simulink model "DNN_x3D_M_2000iA900L_with_6_rev_21a"  (R2021a)
settings: Solver=VariableStepAuto  StartTime=0.0  StopTime=10.0  RelTol=1e-3
model workspace: external: MATLAB File /home/archistrax/Desktop/DNN/Simulink/Brazo robotico (2)/x3D_M_2000iA900L_OLGA_DataFile8.m (data not in the file)
values from neighbouring files (symbols this model uses):
  smiData = struct    [x3D_M_2000iA900L_OLGA_DataFile8.m]
undefined symbols (not defined in the file or in its folder): X, Y, Z
libraries: sm_lib x78, nesl_utility x31, pid_lib x15, dspmtrx3 x4
(part 1 of 4)
settings Model: Creator=olegfilatov  LastModifiedBy=archistrax
settings DataIOCC: InspectSignalLogs=on
settings HardwareCC: ProdBitPerLong=64  ProdHWDeviceType=Intel->x86-64 (Linux 64)

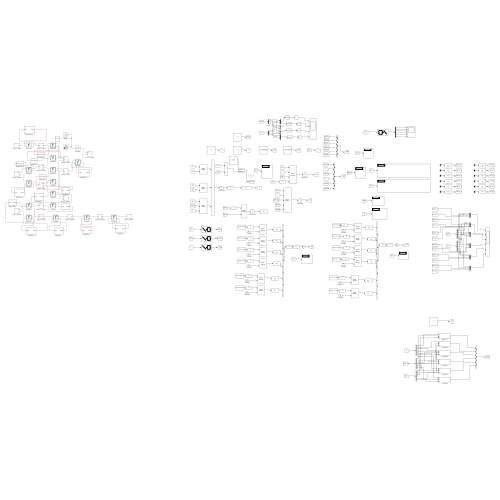
[thumbnail: Simulink's stored preview of the top-level diagram]
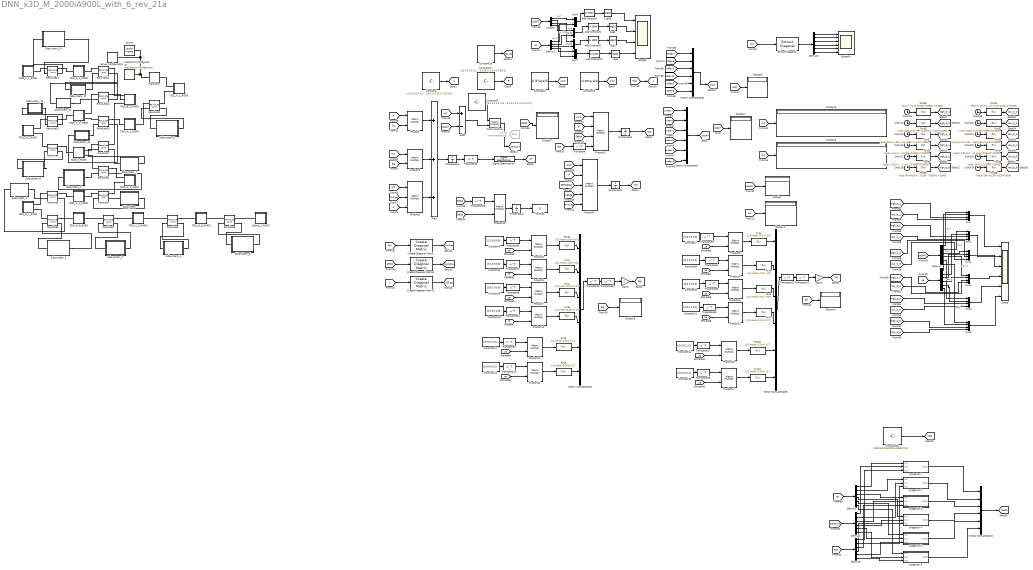
== system DNN_x3D_M_2000iA900L_with_6_rev_21a ==
  " " : Demux  Outputs=6
  Add : Sum  Inputs=+++
  Add Constant{,1..3} (4 alike) : Bias  Bias=1500
  Add1 : Sum  Inputs=+-
  Cabina_2_RIGID : Subsystem
  Clock{13..24} (12 alike) : Clock
  Constant : Constant  Value=[-25 0 0 0 0 0; 0 -35 0 0 0 0; 0 0 -15 0 0 0; 0 0 0 -19 0 0; 0 0 0 0 -20 0; 0 0 0 0 0 -20 ]*5.5  VectorParams1D=off
  Constant1 : Constant  Value=[5 0 0 0 0 0; 0 8 0 0 0 0; 0 0 10 0 0 0; 0 0 0 5 0 0; 0 0 0 0 5 0; 0 0 0 0 0 5 ]
  Constant10 : Constant  Value=[0 0 0 1 0 0]
  Constant11 : Constant  Value=[0 0 0 1 0 0]
  Constant12 : Constant  Value=[0 0 0 0 1 0]
  Constant13 : Constant  Value=[0 0 0 0 0 1]
  Constant14 : Constant  Value=[0 0 0 0 1 0]
  Constant15 : Constant  Value=[0 0 0 0 0 1]
  Constant16 : Constant  Value=[18 1 6 0.2; 1 25 5 0.4; 6 5 12 0.8; 0.2 0.4 0.8 22]*22  VectorParams1D=off
  Constant17 : Constant  Value=[25 0 0 0 0 0; 0 25 0 0 0 0; 0 0 10 0 0 0; 0 0 0 30 0 0; 0 0 0 0 25 0; 0 0 0 0 0 8]*15
  Constant18 : Constant  Value=[950;450;735;2200;40;650]*100
  Constant2 : Constant  Value=-0.8*eye(6)
  Constant3 : Constant  Value=-0.05*eye(6)
  Constant4 : Constant  Value=[1 0 0 0 0 0]
  Constant5 : Constant  Value=[0 1 0 0 0 0]
  Constant6 : Constant  Value=[0 0 1 0 0 0]
  Constant7 : Constant  Value=[1 0 0 0 0 0]
  Constant8 : Constant  Value=[0 1 0 0 0 0]
  Constant9 : Constant  Value=[0 0 1 0 0 0]
  Create Diagonal Matrix : dspmtrx3/Create Diagonal Matrix
      settings: SourceProductBaseCode=SL
  Create Diagonal Matrix1 : dspmtrx3/Create Diagonal Matrix
      settings: SourceProductBaseCode=SL
  Create Diagonal Matrix2 : dspmtrx3/Create Diagonal Matrix
      settings: SourceProductBaseCode=SL
  Demux{1,3..6} (5 alike) : Demux  Outputs=6
  Demux2 : Demux
  Display{,1..8} (9 alike) : Display
  Extract Diagonal : dspmtrx3/Extract Diagonal
      settings: SourceProductBaseCode=SL
  Fcn{1,3..5,11} (5 alike) : Fcn  Expr=2/(1+exp(-2*u))+0.5
  Fcn{2,6..10,12} (7 alike) : Fcn  Expr=1/(1+exp(-0.2*u))-0.7
  Fcn25 : Fcn  Expr=(exp(-u+0.1)+0.03+0.038*u)*10000
  Fcn26 : Fcn  Expr=(exp(-100*u+3)+0.31+0.0299*u-(0.007*u)^(0.5))*10000
  Fcn27 : Fcn  Expr=(exp(-0.2*u-1.05)*(sin(1.88*u)+2.5))*10000
  Fcn28 : Fcn  Expr=(exp(-u+0.1)+0.045+0.032*u)*10000
  Fcn29 : Fcn  Expr=(exp(-1.9*u+1.2)+0.2-0.008*u)*10000
  Fcn30 : Fcn  Expr=(exp(-8*u+6.5)+0.205 - 0.003*u)*10000
  Fcn31 : Fcn  Expr=(-exp(-2.2*u+1.2)-0.14+0.03*u)*10000
  Fcn32 : Fcn  Expr=(-exp(-100*u)-0.043+0.03*u)*10000
  Fcn33 : Fcn  Expr=-(exp(-0.2*u-0.5)*(1.8*cos(1.6*u)+2.8))*10000
  Fcn34 : Fcn  Expr=(-exp(-2.2*u+1.2)-0.14+0.03*u)*10000
  Fcn35 : Fcn  Expr=(-exp(-2*u+1.2)-0.42)*10000
  Fcn36 : Fcn  Expr=-(exp(-10*u+0.9)+0.53)*10000
  Gain3 : Gain
  Gain4 : Gain
  Goto31 : Goto  Commented=on  GotoTag=Delta  TagVisibility=global
  Log{1..3,10} (4 alike) : Math  Operator=log10  SaturateOnIntegerOverflow=on
  Matrix Multiply : Product  Multiplication=Matrix(*)
  MechanismConfiguration : sm_lib/Utilities/Mechanism Configuration  UniformGravity=Constant  GravityVector=[0 -9.80665 0]  GravityUnits=m/s^2  LinearizationDelta=0.001  JointModeTransitionNonlinearIterations=2
  Mux{,1..3,8..9} (6 alike) : Mux
  Mux{4..7} (4 alike) : Mux  Inputs=2
  Ozone-Gas1 : Integrator  InitialCondition=[0.2,0.1,0.01, 0.2,0.1,0.2;0.1,0.6,0.7,0.9,0.2,0.1;0.2,0.2,0.3,0.7,0.1,0.2; 0.2,0.9,0.7,0.5,0.2,0.1;0.1,0.2,0.3,0.4,0.2,0.2;0.4,0.3,0.2,0.1,0.1,0.2]
  Ozone-Gas2 : Integrator  InitialCondition=[0.2,0.1,0.01, 0.2,0.1,0.2;0.1,0.6,0.7,0.9,0.2,0.1;0.2,0.2,0.3,0.7,0.1,0.2; 0.2,0.9,0.7,0.5,0.2,0.1;0.1,0.2,0.3,0.4,0.2,0.2;0.4,0.3,0.2,0.1,0.1,0.2]
  Ozone-Gas3 : Integrator  InitialCondition=[0.2;0.3;0.1;0.3;0.2;0.2]*0.01
  Ozone-Gas4 : Integrator
  Product{,1,5..17} (15 alike) : Product  Multiplication=Matrix(*)
  Product2 : Product  Inputs=3  Multiplication=Matrix(*)
  Product3 : Product  Inputs=4  Multiplication=Matrix(*)
  Product4 : Product  Inputs=5  Multiplication=Matrix(*)
  Revolute : sm_lib/Joints/Revolute Joint  JointMode=Normal  SenseConstraintForce=off  SenseConstraintForceX=off  SenseConstraintForceY=off  SenseConstraintForceZ=off  SenseConstraintTorque=off  SenseConstraintTorqueX=off  SenseConstraintTorqueY=off  SenseConstraintTorqueZ=off  SenseTotalForce=off  SenseTotalForceX=off  SenseTotalForceY=off  SenseTotalForceZ=off  SenseTotalTorque=off  SenseTotalTorqueX=off  SenseTotalTorqueY=off  SenseTotalTorqueZ=off  CompositeWrenchDir=FollowerOnBase  CompositeWrenchFrame=BaseFrame  EquilibriumPosition=0  EquilibriumPositionUnits=deg  SpringStiffness=0  SpringStiffnessUnits=N*m/deg  DampingCoefficient=0  DampingCoefficientUnits=N*m/(deg/s)  TorqueActuationMode=InputTorque  MotionActuationMode=ComputedMotion  SensePosition=on  SenseVelocity=off  SenseAcceleration=off  SenseTorqueForce=off  SenseLowerLimitTorqueForce=off  SenseUpperLimitTorqueForce=off  LowerLimitSpecify=off  LowerLimitBound=-90  LowerLimitBoundUnits=deg  LowerLimitStiffness=1e4  LowerLimitStiffnessUnits=N*m/deg  LowerLimitDamping=10  LowerLimitDampingUnits=N*m/(deg/s)  LowerLimitTransitionRegionWidth=0.1  LowerLimitTransitionRegionWidthUnits=deg  UpperLimitSpecify=off  UpperLimitBound=90  UpperLimitBoundUnits=deg  UpperLimitStiffness=1e4  UpperLimitStiffnessUnits=N*m/deg  UpperLimitDamping=10  UpperLimitDampingUnits=N*m/(deg/s)  UpperLimitTransitionRegionWidth=0.1  UpperLimitTransitionRegionWidthUnits=deg  PositionTargetSpecify=on  PositionTargetPriority=Low  PositionTargetValue=smiData.RevoluteJoint(1).Rz.Pos  PositionTargetValueUnits=deg  VelocityTargetSpecify=off  VelocityTargetPriority=High  VelocityTargetValue=0  VelocityTargetValueUnits=deg/s
  Revolute1 : sm_lib/Joints/Revolute Joint  JointMode=Normal  SenseConstraintForce=off  SenseConstraintForceX=off  SenseConstraintForceY=off  SenseConstraintForceZ=off  SenseConstraintTorque=off  SenseConstraintTorqueX=off  SenseConstraintTorqueY=off  SenseConstraintTorqueZ=off  SenseTotalForce=off  SenseTotalForceX=off  SenseTotalForceY=off  SenseTotalForceZ=off  SenseTotalTorque=off  SenseTotalTorqueX=off  SenseTotalTorqueY=off  SenseTotalTorqueZ=off  CompositeWrenchDir=FollowerOnBase  CompositeWrenchFrame=BaseFrame  EquilibriumPosition=0  EquilibriumPositionUnits=deg  SpringStiffness=0  SpringStiffnessUnits=N*m/deg  DampingCoefficient=0  DampingCoefficientUnits=N*m/(deg/s)  TorqueActuationMode=InputTorque  MotionActuationMode=ComputedMotion  SensePosition=on  SenseVelocity=off  SenseAcceleration=off  SenseTorqueForce=off  SenseLowerLimitTorqueForce=off  SenseUpperLimitTorqueForce=off  LowerLimitSpecify=off  LowerLimitBound=-90  LowerLimitBoundUnits=deg  LowerLimitStiffness=1e4  LowerLimitStiffnessUnits=N*m/deg  LowerLimitDamping=10  LowerLimitDampingUnits=N*m/(deg/s)  LowerLimitTransitionRegionWidth=0.1  LowerLimitTransitionRegionWidthUnits=deg  UpperLimitSpecify=off  UpperLimitBound=90  UpperLimitBoundUnits=deg  UpperLimitStiffness=1e4  UpperLimitStiffnessUnits=N*m/deg  UpperLimitDamping=10  UpperLimitDampingUnits=N*m/(deg/s)  UpperLimitTransitionRegionWidth=0.1  UpperLimitTransitionRegionWidthUnits=deg  PositionTargetSpecify=on  PositionTargetPriority=Low  PositionTargetValue=smiData.RevoluteJoint(2).Rz.Pos  PositionTargetValueUnits=deg  VelocityTargetSpecify=off  VelocityTargetPriority=High  VelocityTargetValue=0  VelocityTargetValueUnits=deg/s
  Revolute10 : sm_lib/Joints/Revolute Joint  JointMode=Normal  SenseConstraintForce=off  SenseConstraintForceX=off  SenseConstraintForceY=off  SenseConstraintForceZ=off  SenseConstraintTorque=off  SenseConstraintTorqueX=off  SenseConstraintTorqueY=off  SenseConstraintTorqueZ=off  SenseTotalForce=off  SenseTotalForceX=off  SenseTotalForceY=off  SenseTotalForceZ=off  SenseTotalTorque=off  SenseTotalTorqueX=off  SenseTotalTorqueY=off  SenseTotalTorqueZ=off  CompositeWrenchDir=FollowerOnBase  CompositeWrenchFrame=BaseFrame  EquilibriumPosition=0  EquilibriumPositionUnits=deg  SpringStiffness=0  SpringStiffnessUnits=N*m/deg  DampingCoefficient=0  DampingCoefficientUnits=N*m/(deg/s)  TorqueActuationMode=InputTorque  MotionActuationMode=ComputedMotion  SensePosition=on  SenseVelocity=off  SenseAcceleration=off  SenseTorqueForce=off  SenseLowerLimitTorqueForce=off  SenseUpperLimitTorqueForce=off  LowerLimitSpecify=off  LowerLimitBound=-90  LowerLimitBoundUnits=deg  LowerLimitStiffness=1e4  LowerLimitStiffnessUnits=N*m/deg  LowerLimitDamping=10  LowerLimitDampingUnits=N*m/(deg/s)  LowerLimitTransitionRegionWidth=0.1  LowerLimitTransitionRegionWidthUnits=deg  UpperLimitSpecify=off  UpperLimitBound=90  UpperLimitBoundUnits=deg  UpperLimitStiffness=1e4  UpperLimitStiffnessUnits=N*m/deg  UpperLimitDamping=10  UpperLimitDampingUnits=N*m/(deg/s)  UpperLimitTransitionRegionWidth=0.1  UpperLimitTransitionRegionWidthUnits=deg  PositionTargetSpecify=on  PositionTargetPriority=Low  PositionTargetValue=smiData.RevoluteJoint(11).Rz.Pos  PositionTargetValueUnits=deg  VelocityTargetSpecify=off  VelocityTargetPriority=High  VelocityTargetValue=0  VelocityTargetValueUnits=deg/s
  Revolute11 : sm_lib/Joints/Revolute Joint  JointMode=Normal  SenseConstraintForce=off  SenseConstraintForceX=off  SenseConstraintForceY=off  SenseConstraintForceZ=off  SenseConstraintTorque=off  SenseConstraintTorqueX=off  SenseConstraintTorqueY=off  SenseConstraintTorqueZ=off  SenseTotalForce=off  SenseTotalForceX=off  SenseTotalForceY=off  SenseTotalForceZ=off  SenseTotalTorque=off  SenseTotalTorqueX=off  SenseTotalTorqueY=off  SenseTotalTorqueZ=off  CompositeWrenchDir=FollowerOnBase  CompositeWrenchFrame=BaseFrame  EquilibriumPosition=0  EquilibriumPositionUnits=deg  SpringStiffness=0  SpringStiffnessUnits=N*m/deg  DampingCoefficient=0  DampingCoefficientUnits=N*m/(deg/s)  TorqueActuationMode=InputTorque  MotionActuationMode=ComputedMotion  SensePosition=on  SenseVelocity=off  SenseAcceleration=off  SenseTorqueForce=off  SenseLowerLimitTorqueForce=off  SenseUpperLimitTorqueForce=off  LowerLimitSpecify=off  LowerLimitBound=-90  LowerLimitBoundUnits=deg  LowerLimitStiffness=1e4  LowerLimitStiffnessUnits=N*m/deg  LowerLimitDamping=10  LowerLimitDampingUnits=N*m/(deg/s)  LowerLimitTransitionRegionWidth=0.1  LowerLimitTransitionRegionWidthUnits=deg  UpperLimitSpecify=off  UpperLimitBound=90  UpperLimitBoundUnits=deg  UpperLimitStiffness=1e4  UpperLimitStiffnessUnits=N*m/deg  UpperLimitDamping=10  UpperLimitDampingUnits=N*m/(deg/s)  UpperLimitTransitionRegionWidth=0.1  UpperLimitTransitionRegionWidthUnits=deg  PositionTargetSpecify=on  PositionTargetPriority=Low  PositionTargetValue=smiData.RevoluteJoint(12).Rz.Pos  PositionTargetValueUnits=deg  VelocityTargetSpecify=off  VelocityTargetPriority=High  VelocityTargetValue=0  VelocityTargetValueUnits=deg/s
  Revolute12 : sm_lib/Joints/Revolute Joint  JointMode=Normal  SenseConstraintForce=off  SenseConstraintForceX=off  SenseConstraintForceY=off  SenseConstraintForceZ=off  SenseConstraintTorque=off  SenseConstraintTorqueX=off  SenseConstraintTorqueY=off  SenseConstraintTorqueZ=off  SenseTotalForce=off  SenseTotalForceX=off  SenseTotalForceY=off  SenseTotalForceZ=off  SenseTotalTorque=off  SenseTotalTorqueX=off  SenseTotalTorqueY=off  SenseTotalTorqueZ=off  CompositeWrenchDir=FollowerOnBase  CompositeWrenchFrame=BaseFrame  EquilibriumPosition=0  EquilibriumPositionUnits=deg  SpringStiffness=0  SpringStiffnessUnits=N*m/deg  DampingCoefficient=0  DampingCoefficientUnits=N*m/(deg/s)  TorqueActuationMode=InputTorque  MotionActuationMode=ComputedMotion  SensePosition=on  SenseVelocity=off  SenseAcceleration=off  SenseTorqueForce=off  SenseLowerLimitTorqueForce=off  SenseUpperLimitTorqueForce=off  LowerLimitSpecify=on  LowerLimitBound=-60  LowerLimitBoundUnits=deg  LowerLimitStiffness=1e4  LowerLimitStiffnessUnits=N*m/deg  LowerLimitDamping=10  LowerLimitDampingUnits=N*m/(deg/s)  LowerLimitTransitionRegionWidth=0.1  LowerLimitTransitionRegionWidthUnits=deg  UpperLimitSpecify=on  UpperLimitBound=100  UpperLimitBoundUnits=deg  UpperLimitStiffness=1e4  UpperLimitStiffnessUnits=N*m/deg  UpperLimitDamping=10  UpperLimitDampingUnits=N*m/(deg/s)  UpperLimitTransitionRegionWidth=0.1  UpperLimitTransitionRegionWidthUnits=deg  PositionTargetSpecify=on  PositionTargetPriority=Low  PositionTargetValue=smiData.RevoluteJoint(13).Rz.Pos  PositionTargetValueUnits=deg  VelocityTargetSpecify=off  VelocityTargetPriority=High  VelocityTargetValue=0  VelocityTargetValueUnits=deg/s
  Revolute13 : sm_lib/Joints/Revolute Joint  JointMode=Normal  SenseConstraintForce=off  SenseConstraintForceX=off  SenseConstraintForceY=off  SenseConstraintForceZ=off  SenseConstraintTorque=off  SenseConstraintTorqueX=off  SenseConstraintTorqueY=off  SenseConstraintTorqueZ=off  SenseTotalForce=off  SenseTotalForceX=off  SenseTotalForceY=off  SenseTotalForceZ=off  SenseTotalTorque=off  SenseTotalTorqueX=off  SenseTotalTorqueY=off  SenseTotalTorqueZ=off  CompositeWrenchDir=FollowerOnBase  CompositeWrenchFrame=BaseFrame  EquilibriumPosition=0  EquilibriumPositionUnits=deg  SpringStiffness=0  SpringStiffnessUnits=N*m/deg  DampingCoefficient=0  DampingCoefficientUnits=N*m/(deg/s)  TorqueActuationMode=InputTorque  MotionActuationMode=ComputedMotion  SensePosition=on  SenseVelocity=off  SenseAcceleration=off  SenseTorqueForce=off  SenseLowerLimitTorqueForce=off  SenseUpperLimitTorqueForce=off  LowerLimitSpecify=off  LowerLimitBound=-90  LowerLimitBoundUnits=deg  LowerLimitStiffness=1e4  LowerLimitStiffnessUnits=N*m/deg  LowerLimitDamping=10  LowerLimitDampingUnits=N*m/(deg/s)  LowerLimitTransitionRegionWidth=0.1  LowerLimitTransitionRegionWidthUnits=deg  UpperLimitSpecify=off  UpperLimitBound=90  UpperLimitBoundUnits=deg  UpperLimitStiffness=1e4  UpperLimitStiffnessUnits=N*m/deg  UpperLimitDamping=10  UpperLimitDampingUnits=N*m/(deg/s)  UpperLimitTransitionRegionWidth=0.1  UpperLimitTransitionRegionWidthUnits=deg  PositionTargetSpecify=on  PositionTargetPriority=Low  PositionTargetValue=smiData.RevoluteJoint(14).Rz.Pos  PositionTargetValueUnits=deg  VelocityTargetSpecify=off  VelocityTargetPriority=High  VelocityTargetValue=0  VelocityTargetValueUnits=deg/s
  Revolute14 : sm_lib/Joints/Revolute Joint  JointMode=Normal  SenseConstraintForce=off  SenseConstraintForceX=off  SenseConstraintForceY=off  SenseConstraintForceZ=off  SenseConstraintTorque=off  SenseConstraintTorqueX=off  SenseConstraintTorqueY=off  SenseConstraintTorqueZ=off  SenseTotalForce=off  SenseTotalForceX=off  SenseTotalForceY=off  SenseTotalForceZ=off  SenseTotalTorque=off  SenseTotalTorqueX=off  SenseTotalTorqueY=off  SenseTotalTorqueZ=off  CompositeWrenchDir=FollowerOnBase  CompositeWrenchFrame=BaseFrame  EquilibriumPosition=0  EquilibriumPositionUnits=deg  SpringStiffness=0  SpringStiffnessUnits=N*m/deg  DampingCoefficient=0  DampingCoefficientUnits=N*m/(deg/s)  TorqueActuationMode=InputTorque  MotionActuationMode=ComputedMotion  SensePosition=on  SenseVelocity=off  SenseAcceleration=off  SenseTorqueForce=off  SenseLowerLimitTorqueForce=off  SenseUpperLimitTorqueForce=off  LowerLimitSpecify=off  LowerLimitBound=-90  LowerLimitBoundUnits=deg  LowerLimitStiffness=1e4  LowerLimitStiffnessUnits=N*m/deg  LowerLimitDamping=10  LowerLimitDampingUnits=N*m/(deg/s)  LowerLimitTransitionRegionWidth=0.1  LowerLimitTransitionRegionWidthUnits=deg  UpperLimitSpecify=off  UpperLimitBound=90  UpperLimitBoundUnits=deg  UpperLimitStiffness=1e4  UpperLimitStiffnessUnits=N*m/deg  UpperLimitDamping=10  UpperLimitDampingUnits=N*m/(deg/s)  UpperLimitTransitionRegionWidth=0.1  UpperLimitTransitionRegionWidthUnits=deg  PositionTargetSpecify=on  PositionTargetPriority=Low  PositionTargetValue=smiData.RevoluteJoint(15).Rz.Pos  PositionTargetValueUnits=deg  VelocityTargetSpecify=off  VelocityTargetPriority=High  VelocityTargetValue=0  VelocityTargetValueUnits=deg/s
  Revolute2 : sm_lib/Joints/Revolute Joint  JointMode=Normal  SenseConstraintForce=off  SenseConstraintForceX=off  SenseConstraintForceY=off  SenseConstraintForceZ=off  SenseConstraintTorque=off  SenseConstraintTorqueX=off  SenseConstraintTorqueY=off  SenseConstraintTorqueZ=off  SenseTotalForce=off  SenseTotalForceX=off  SenseTotalForceY=off  SenseTotalForceZ=off  SenseTotalTorque=off  SenseTotalTorqueX=off  SenseTotalTorqueY=off  SenseTotalTorqueZ=off  CompositeWrenchDir=FollowerOnBase  CompositeWrenchFrame=BaseFrame  EquilibriumPosition=0  EquilibriumPositionUnits=deg  SpringStiffness=0  SpringStiffnessUnits=N*m/deg  DampingCoefficient=0  DampingCoefficientUnits=N*m/(deg/s)  TorqueActuationMode=InputTorque  MotionActuationMode=ComputedMotion  SensePosition=on  SenseVelocity=off  SenseAcceleration=off  SenseTorqueForce=off  SenseLowerLimitTorqueForce=off  SenseUpperLimitTorqueForce=off  LowerLimitSpecify=on  LowerLimitBound=-120  LowerLimitBoundUnits=deg  LowerLimitStiffness=1e4  LowerLimitStiffnessUnits=N*m/deg  LowerLimitDamping=10  LowerLimitDampingUnits=N*m/(deg/s)  LowerLimitTransitionRegionWidth=0.1  LowerLimitTransitionRegionWidthUnits=deg  UpperLimitSpecify=on  UpperLimitBound=120  UpperLimitBoundUnits=deg  UpperLimitStiffness=1e4  UpperLimitStiffnessUnits=N*m/deg  UpperLimitDamping=10  UpperLimitDampingUnits=N*m/(deg/s)  UpperLimitTransitionRegionWidth=0.1  UpperLimitTransitionRegionWidthUnits=deg  PositionTargetSpecify=on  PositionTargetPriority=Low  PositionTargetValue=smiData.RevoluteJoint(3).Rz.Pos  PositionTargetValueUnits=deg  VelocityTargetSpecify=off  VelocityTargetPriority=High  VelocityTargetValue=0  VelocityTargetValueUnits=deg/s
  Revolute3 : sm_lib/Joints/Revolute Joint  JointMode=Normal  SenseConstraintForce=off  SenseConstraintForceX=off  SenseConstraintForceY=off  SenseConstraintForceZ=off  SenseConstraintTorque=off  SenseConstraintTorqueX=off  SenseConstraintTorqueY=off  SenseConstraintTorqueZ=off  SenseTotalForce=off  SenseTotalForceX=off  SenseTotalForceY=off  SenseTotalForceZ=off  SenseTotalTorque=off  SenseTotalTorqueX=off  SenseTotalTorqueY=off  SenseTotalTorqueZ=off  CompositeWrenchDir=FollowerOnBase  CompositeWrenchFrame=BaseFrame  EquilibriumPosition=0  EquilibriumPositionUnits=deg  SpringStiffness=0  SpringStiffnessUnits=N*m/deg  DampingCoefficient=0  DampingCoefficientUnits=N*m/(deg/s)  TorqueActuationMode=InputTorque  MotionActuationMode=ComputedMotion  SensePosition=on  SenseVelocity=off  SenseAcceleration=off  SenseTorqueForce=off  SenseLowerLimitTorqueForce=off  SenseUpperLimitTorqueForce=off  LowerLimitSpecify=on  LowerLimitBound=-360  LowerLimitBoundUnits=deg  LowerLimitStiffness=1e4  LowerLimitStiffnessUnits=N*m/deg  LowerLimitDamping=10  LowerLimitDampingUnits=N*m/(deg/s)  LowerLimitTransitionRegionWidth=0.1  LowerLimitTransitionRegionWidthUnits=deg  UpperLimitSpecify=on  UpperLimitBound=360  UpperLimitBoundUnits=deg  UpperLimitStiffness=1e4  UpperLimitStiffnessUnits=N*m/deg  UpperLimitDamping=10  UpperLimitDampingUnits=N*m/(deg/s)  UpperLimitTransitionRegionWidth=0.1  UpperLimitTransitionRegionWidthUnits=deg  PositionTargetSpecify=on  PositionTargetPriority=Low  PositionTargetValue=smiData.RevoluteJoint(4).Rz.Pos  PositionTargetValueUnits=deg  VelocityTargetSpecify=off  VelocityTargetPriority=High  VelocityTargetValue=0  VelocityTargetValueUnits=deg/s
  Revolute4 : sm_lib/Joints/Revolute Joint  JointMode=Normal  SenseConstraintForce=off  SenseConstraintForceX=off  SenseConstraintForceY=off  SenseConstraintForceZ=off  SenseConstraintTorque=off  SenseConstraintTorqueX=off  SenseConstraintTorqueY=off  SenseConstraintTorqueZ=off  SenseTotalForce=off  SenseTotalForceX=off  SenseTotalForceY=off  SenseTotalForceZ=off  SenseTotalTorque=off  SenseTotalTorqueX=off  SenseTotalTorqueY=off  SenseTotalTorqueZ=off  CompositeWrenchDir=FollowerOnBase  CompositeWrenchFrame=BaseFrame  EquilibriumPosition=0  EquilibriumPositionUnits=deg  SpringStiffness=0  SpringStiffnessUnits=N*m/deg  DampingCoefficient=0  DampingCoefficientUnits=N*m/(deg/s)  TorqueActuationMode=InputTorque  MotionActuationMode=ComputedMotion  SensePosition=on  SenseVelocity=off  SenseAcceleration=off  SenseTorqueForce=off  SenseLowerLimitTorqueForce=off  SenseUpperLimitTorqueForce=off  LowerLimitSpecify=off  LowerLimitBound=-90  LowerLimitBoundUnits=deg  LowerLimitStiffness=1e4  LowerLimitStiffnessUnits=N*m/deg  LowerLimitDamping=10  LowerLimitDampingUnits=N*m/(deg/s)  LowerLimitTransitionRegionWidth=0.1  LowerLimitTransitionRegionWidthUnits=deg  UpperLimitSpecify=off  UpperLimitBound=90  UpperLimitBoundUnits=deg  UpperLimitStiffness=1e4  UpperLimitStiffnessUnits=N*m/deg  UpperLimitDamping=10  UpperLimitDampingUnits=N*m/(deg/s)  UpperLimitTransitionRegionWidth=0.1  UpperLimitTransitionRegionWidthUnits=deg  PositionTargetSpecify=on  PositionTargetPriority=Low  PositionTargetValue=smiData.RevoluteJoint(5).Rz.Pos  PositionTargetValueUnits=deg  VelocityTargetSpecify=off  VelocityTargetPriority=High  VelocityTargetValue=0  VelocityTargetValueUnits=deg/s
  Revolute5 : sm_lib/Joints/Revolute Joint  JointMode=Normal  SenseConstraintForce=off  SenseConstraintForceX=off  SenseConstraintForceY=off  SenseConstraintForceZ=off  SenseConstraintTorque=off  SenseConstraintTorqueX=off  SenseConstraintTorqueY=off  SenseConstraintTorqueZ=off  SenseTotalForce=off  SenseTotalForceX=off  SenseTotalForceY=off  SenseTotalForceZ=off  SenseTotalTorque=off  SenseTotalTorqueX=off  SenseTotalTorqueY=off  SenseTotalTorqueZ=off  CompositeWrenchDir=FollowerOnBase  CompositeWrenchFrame=BaseFrame  EquilibriumPosition=0  EquilibriumPositionUnits=deg  SpringStiffness=0  SpringStiffnessUnits=N*m/deg  DampingCoefficient=0  DampingCoefficientUnits=N*m/(deg/s)  TorqueActuationMode=InputTorque  MotionActuationMode=ComputedMotion  SensePosition=on  SenseVelocity=off  SenseAcceleration=off  SenseTorqueForce=off  SenseLowerLimitTorqueForce=off  SenseUpperLimitTorqueForce=off  LowerLimitSpecify=off  LowerLimitBound=-90  LowerLimitBoundUnits=deg  LowerLimitStiffness=1e4  LowerLimitStiffnessUnits=N*m/deg  LowerLimitDamping=10  LowerLimitDampingUnits=N*m/(deg/s)  LowerLimitTransitionRegionWidth=0.1  LowerLimitTransitionRegionWidthUnits=deg  UpperLimitSpecify=off  UpperLimitBound=90  UpperLimitBoundUnits=deg  UpperLimitStiffness=1e4  UpperLimitStiffnessUnits=N*m/deg  UpperLimitDamping=10  UpperLimitDampingUnits=N*m/(deg/s)  UpperLimitTransitionRegionWidth=0.1  UpperLimitTransitionRegionWidthUnits=deg  PositionTargetSpecify=on  PositionTargetPriority=Low  PositionTargetValue=smiData.RevoluteJoint(6).Rz.Pos  PositionTargetValueUnits=deg  VelocityTargetSpecify=off  VelocityTargetPriority=High  VelocityTargetValue=0  VelocityTargetValueUnits=deg/s
  Revolute6 : sm_lib/Joints/Revolute Joint  JointMode=Normal  SenseConstraintForce=off  SenseConstraintForceX=off  SenseConstraintForceY=off  SenseConstraintForceZ=off  SenseConstraintTorque=off  SenseConstraintTorqueX=off  SenseConstraintTorqueY=off  SenseConstraintTorqueZ=off  SenseTotalForce=off  SenseTotalForceX=off  SenseTotalForceY=off  SenseTotalForceZ=off  SenseTotalTorque=off  SenseTotalTorqueX=off  SenseTotalTorqueY=off  SenseTotalTorqueZ=off  CompositeWrenchDir=FollowerOnBase  CompositeWrenchFrame=BaseFrame  EquilibriumPosition=0  EquilibriumPositionUnits=deg  SpringStiffness=0  SpringStiffnessUnits=N*m/deg  DampingCoefficient=0  DampingCoefficientUnits=N*m/(deg/s)  TorqueActuationMode=InputTorque  MotionActuationMode=ComputedMotion  SensePosition=on  SenseVelocity=off  SenseAcceleration=off  SenseTorqueForce=off  SenseLowerLimitTorqueForce=off  SenseUpperLimitTorqueForce=off  LowerLimitSpecify=on  LowerLimitBound=-360  LowerLimitBoundUnits=deg  LowerLimitStiffness=1e4  LowerLimitStiffnessUnits=N*m/deg  LowerLimitDamping=10  LowerLimitDampingUnits=N*m/(deg/s)  LowerLimitTransitionRegionWidth=0.1  LowerLimitTransitionRegionWidthUnits=deg  UpperLimitSpecify=on  UpperLimitBound=360  UpperLimitBoundUnits=deg  UpperLimitStiffness=1e4  UpperLimitStiffnessUnits=N*m/deg  UpperLimitDamping=10  UpperLimitDampingUnits=N*m/(deg/s)  UpperLimitTransitionRegionWidth=0.1  UpperLimitTransitionRegionWidthUnits=deg  PositionTargetSpecify=on  PositionTargetPriority=Low  PositionTargetValue=smiData.RevoluteJoint(7).Rz.Pos  PositionTargetValueUnits=deg  VelocityTargetSpecify=off  VelocityTargetPriority=High  VelocityTargetValue=0  VelocityTargetValueUnits=deg/s
  Revolute7 : sm_lib/Joints/Revolute Joint  JointMode=Normal  SenseConstraintForce=off  SenseConstraintForceX=off  SenseConstraintForceY=off  SenseConstraintForceZ=off  SenseConstraintTorque=off  SenseConstraintTorqueX=off  SenseConstraintTorqueY=off  SenseConstraintTorqueZ=off  SenseTotalForce=off  SenseTotalForceX=off  SenseTotalForceY=off  SenseTotalForceZ=off  SenseTotalTorque=off  SenseTotalTorqueX=off  SenseTotalTorqueY=off  SenseTotalTorqueZ=off  CompositeWrenchDir=FollowerOnBase  CompositeWrenchFrame=BaseFrame  EquilibriumPosition=0  EquilibriumPositionUnits=deg  SpringStiffness=0  SpringStiffnessUnits=N*m/deg  DampingCoefficient=0  DampingCoefficientUnits=N*m/(deg/s)  TorqueActuationMode=InputTorque  MotionActuationMode=ComputedMotion  SensePosition=on  SenseVelocity=off  SenseAcceleration=off  SenseTorqueForce=off  SenseLowerLimitTorqueForce=off  SenseUpperLimitTorqueForce=off  LowerLimitSpecify=on  LowerLimitBound=-130  LowerLimitBoundUnits=deg  LowerLimitStiffness=1e4  LowerLimitStiffnessUnits=N*m/deg  LowerLimitDamping=10  LowerLimitDampingUnits=N*m/(deg/s)  LowerLimitTransitionRegionWidth=0.1  LowerLimitTransitionRegionWidthUnits=deg  UpperLimitSpecify=on  UpperLimitBound=35  UpperLimitBoundUnits=deg  UpperLimitStiffness=1e4  UpperLimitStiffnessUnits=N*m/deg  UpperLimitDamping=10  UpperLimitDampingUnits=N*m/(deg/s)  UpperLimitTransitionRegionWidth=0.1  UpperLimitTransitionRegionWidthUnits=deg  PositionTargetSpecify=on  PositionTargetPriority=Low  PositionTargetValue=smiData.RevoluteJoint(8).Rz.Pos  PositionTargetValueUnits=deg  VelocityTargetSpecify=off  VelocityTargetPriority=High  VelocityTargetValue=0  VelocityTargetValueUnits=deg/s
  Revolute8 : sm_lib/Joints/Revolute Joint  JointMode=Normal  SenseConstraintForce=off  SenseConstraintForceX=off  SenseConstraintForceY=off  SenseConstraintForceZ=off  SenseConstraintTorque=off  SenseConstraintTorqueX=off  SenseConstraintTorqueY=off  SenseConstraintTorqueZ=off  SenseTotalForce=off  SenseTotalForceX=off  SenseTotalForceY=off  SenseTotalForceZ=off  SenseTotalTorque=off  SenseTotalTorqueX=off  SenseTotalTorqueY=off  SenseTotalTorqueZ=off  CompositeWrenchDir=FollowerOnBase  CompositeWrenchFrame=BaseFrame  EquilibriumPosition=0  EquilibriumPositionUnits=deg  SpringStiffness=0  SpringStiffnessUnits=N*m/deg  DampingCoefficient=0  DampingCoefficientUnits=N*m/(deg/s)  TorqueActuationMode=InputTorque  MotionActuationMode=ComputedMotion  SensePosition=on  SenseVelocity=off  SenseAcceleration=off  SenseTorqueForce=off  SenseLowerLimitTorqueForce=off  SenseUpperLimitTorqueForce=off  LowerLimitSpecify=off  LowerLimitBound=-90  LowerLimitBoundUnits=deg  LowerLimitStiffness=1e4  LowerLimitStiffnessUnits=N*m/deg  LowerLimitDamping=10  LowerLimitDampingUnits=N*m/(deg/s)  LowerLimitTransitionRegionWidth=0.1  LowerLimitTransitionRegionWidthUnits=deg  UpperLimitSpecify=off  UpperLimitBound=90  UpperLimitBoundUnits=deg  UpperLimitStiffness=1e4  UpperLimitStiffnessUnits=N*m/deg  UpperLimitDamping=10  UpperLimitDampingUnits=N*m/(deg/s)  UpperLimitTransitionRegionWidth=0.1  UpperLimitTransitionRegionWidthUnits=deg  PositionTargetSpecify=off  PositionTargetPriority=High  PositionTargetValue=0  PositionTargetValueUnits=deg  VelocityTargetSpecify=off  VelocityTargetPriority=High  VelocityTargetValue=0  VelocityTargetValueUnits=deg/s
  Revolute9 : sm_lib/Joints/Revolute Joint  JointMode=Normal  SenseConstraintForce=off  SenseConstraintForceX=off  SenseConstraintForceY=off  SenseConstraintForceZ=off  SenseConstraintTorque=off  SenseConstraintTorqueX=off  SenseConstraintTorqueY=off  SenseConstraintTorqueZ=off  SenseTotalForce=off  SenseTotalForceX=off  SenseTotalForceY=off  SenseTotalForceZ=off  SenseTotalTorque=off  SenseTotalTorqueX=off  SenseTotalTorqueY=off  SenseTotalTorqueZ=off  CompositeWrenchDir=FollowerOnBase  CompositeWrenchFrame=BaseFrame  EquilibriumPosition=0  EquilibriumPositionUnits=deg  SpringStiffness=0  SpringStiffnessUnits=N*m/deg  DampingCoefficient=0  DampingCoefficientUnits=N*m/(deg/s)  TorqueActuationMode=InputTorque  MotionActuationMode=ComputedMotion  SensePosition=on  SenseVelocity=off  SenseAcceleration=off  SenseTorqueForce=off  SenseLowerLimitTorqueForce=off  SenseUpperLimitTorqueForce=off  LowerLimitSpecify=on  LowerLimitBound=-165  LowerLimitBoundUnits=deg  LowerLimitStiffness=1e4  LowerLimitStiffnessUnits=N*m/deg  LowerLimitDamping=10  LowerLimitDampingUnits=N*m/(deg/s)  LowerLimitTransitionRegionWidth=0.1  LowerLimitTransitionRegionWidthUnits=deg  UpperLimitSpecify=on  UpperLimitBound=165  UpperLimitBoundUnits=deg  UpperLimitStiffness=1e4  UpperLimitStiffnessUnits=N*m/deg  UpperLimitDamping=10  UpperLimitDampingUnits=N*m/(deg/s)  UpperLimitTransitionRegionWidth=0.1  UpperLimitTransitionRegionWidthUnits=deg  PositionTargetSpecify=on  PositionTargetPriority=Low  PositionTargetValue=smiData.RevoluteJoint(10).Rz.Pos  PositionTargetValueUnits=deg  VelocityTargetSpecify=off  VelocityTargetPriority=High  VelocityTargetValue=0  VelocityTargetValueUnits=deg/s
  Scope : Scope  NumInputPorts=6
  Scope1 : Scope  NumInputPorts=4
  Scope14 : Scope  NumInputPorts=6
  Signal Specification : SignalSpecification  Dimensions=6
  Solver Configuration : nesl_utility/Solver Configuration  PhysicalDomain=network_engine_domain  SubClassName=solver  LeftPortType=input  RightPortType=generic  Tones=[]  Harmonics=[]  SimulateNoise=off  Profile=off  UseLocalSampling=off  EnableSwitchedLinearOptims=on  FrequencyDomain=off  UseCCode=off  RelTol=0.001  AbsTol=1e-06  MinStep=1e-09  ToWorkspace=off  RevertToSquareIcSolve=off  NumHomotopyIterations=100  PhasorMode=off  PhasorModeNumHarmonics=1  IndexReductionMethod=DerivativeReplacement  DoDC=off  ResidualTolerance=1e-09  UseLocalSolver=off  LocalSolverChoice=NE_BACKWARD_EULER_ADVANCER  LocalSolverSampleTime=0.001  DoFixedCost=off  MaxNonlinIter=3  MaxModeIter=2  ComputeImpulses=off  ImpulseIterations=2  LinearAlgebra=auto  LinearAlgebraNumThread=0  EquationFormulation=NE_TIME_EF  DelaysMemoryBudget=1024  AutomaticFiltering=on  FilteringTimeConstant=0.001  PartitionStorageMethod=AS_NEEDED  PartitionMemoryBudget=1024  PartitionMethod=ROBUST
      settings: SourceProductBaseCode=SS,PW,VE
  Subsystem : Subsystem
  Subsystem_1 : Subsystem
  Subsystem_10 : Subsystem
  Subsystem_11 : Subsystem
  Subsystem_12 : Subsystem
  Subsystem_13 : Subsystem
  Subsystem_14 : Subsystem
  Subsystem_2 : Subsystem
  Subsystem_3 : Subsystem
  Subsystem_4 : Subsystem
  Subsystem_5 : Subsystem
  Subsystem_6 : Subsystem
  Subsystem_7 : Subsystem
  Subsystem_8 : Subsystem
  Subsystem_9 : Subsystem
  T201_A_1_RIGID : Subsystem
  T301_A_1_RIGID : Subsystem
  T301_B_1_RIGID : Subsystem
  T301_D_1_RIGID : Subsystem
  T301_E_1_RIGID : Subsystem
  T301_F_1_RIGID : Subsystem
  T303_C_1_RIGID : Subsystem
  T403_1_RIGID : Subsystem
  T501_A_1_RIGID : Subsystem
  T501_A_6_RIGID : Subsystem
  T501_C_1_RIGID : Subsystem
  T501_C_6_RIGID : Subsystem
  T501_D_1_RIGID : Subsystem
  T501_D_6_RIGID : Subsystem
  To File4 : ToFile  Filename=Q  MatrixName=Q  SaveFormat=Timeseries
  Transform : sm_lib/Frames and Transforms/Rigid Transform  TranslationMethod=Cartesian  TranslationStandardOffset=0  TranslationLengthUnit=mm  TranslationStandardAxis=+Z  TranslationCartesianOffset=smiData.RigidTransform(31).translation  TranslationROffset=0  TranslationROffsetUnits=m  TranslationZOffset=0  TranslationZOffsetUnits=m  TranslationThetaOffset=0  TranslationThetaOffsetUnits=deg  RotationMethod=ArbitraryAxis  RotationAngleUnits=rad  RotationStandardAxis=+Z  RotationAngle=smiData.RigidTransform(31).angle  RotationArbitraryAxis=smiData.RigidTransform(31).axis  FollAlignAxisA=+X  BaseAlignAxisA=+Y  FollAlignAxisB=+Y  BaseAlignAxisB=+Z  RotationSequenceAxes=FollowerAxes  RotationSequence=XYX  RotationSequenceAngles=[0 0 0]  RotationSequenceAnglesUnits=deg  RotationMatrix=[1 0 0; 0 1 0; 0 0 1]
  Transpose{,1..18} (19 alike) : Math  Operator=transpose  SignedPower=on  SaturateOnIntegerOverflow=on
  Vector Concatenate{,1..4} (5 alike) : Concatenate  NumInputs=6
  World : sm_lib/Frames and Transforms/World Frame
  outAll1 : Demux
  progector 2 : Subsystem
  progector 3 : Subsystem
  progector 4 : Subsystem
  progector 5 : Subsystem
  progector 6 : Subsystem
  projector 1 : Subsystem
  tag scope: A=global, Delta=global, DeltaDiag=global, Delta_old=global, P=global, Phi=global, PhiDiag=global, Sig=global, UDiag=global, W1=global, W2=global, eps=global, high_b_1=global, high_b_2=global, high_b_3=global, high_b_4=global, high_b_5=global, high_b_6=global, inAll=global, kw1=global, kw2=global, low_b_1=global, low_b_2=global, low_b_3=global, low_b_4=global, low_b_5=global, low_b_6=global, outAll=global, u=global, xe=global
  wires:
  [outRev7] -> Vector Concatenate/1
  [outRev9] -> Vector Concatenate/2
  [outRev2] -> Vector Concatenate/3
  [outRev12] -> Vector Concatenate/4
  Vector Concatenate/1 -> [outAll]
  [outAll] -> Display1/1
  Vector Concatenate3/1 -> Transpose12/1
  Constant6/1 -> Transpose8/1
  [kw2] -> Product4/1
  [DeltaDiag] -> Product4/3
  [xe] -> Display2/1
  Constant17/1 -> [P]
  Constant10/1 -> Transpose14/1
  Product9/1 -> Fcn3/1
  Fcn1/1 -> Vector Concatenate2/2
  [Phi] -> Display4/1
  Product11/1 -> Fcn6/1
  Fcn3/1 -> Vector Concatenate3/2
  Transpose/1 -> Product3/4
  Constant11/1 -> Transpose15/1
  Transpose9/1 -> Transpose10/1
  [xe] -> Product12/2
  Fcn7/1 -> Vector Concatenate3/4
  [xe] -> Product7/2
  [kw1] -> Product3/1
  Transpose14/1 -> Product11/1
  Vector Concatenate2/1 -> Transpose9/1
  Transpose3/1 -> Product8/1
  Fcn11/1 -> Vector Concatenate2/1
  [inAll] -> [u]
  [W1] -> Product1/1
  Constant5/1 -> Transpose7/1
  [Sig] -> Product1/2
  Transpose5/1 -> Product10/1
  Gain3/1 -> [Sig]
  Gain4/1 -> [Phi]
  Constant7/1 -> Transpose3/1
  [outAll] -> Add1/2
  Product3/1 -> Ozone-Gas1/1
  Fcn5/1 -> Vector Concatenate3/3
  Fcn6/1 -> Vector Concatenate2/4
  Product12/1 -> Fcn7/1
  [W2] -> Product2/1
  Fcn2/1 -> Vector Concatenate2/3
  Transpose2/1 -> Signal Specification/1
  [Delta] -> Product3/3
  [xe] -> Product11/2
  Ozone-Gas3/1 -> Transpose2/1
  [xe] -> Product/2
  Fcn4/1 -> Vector Concatenate3/1
  [P] -> Product4/2
  [PhiDiag] -> Product2/2
  [Sig] -> Display3/1
  Transpose12/1 -> Transpose11/1
  Transpose6/1 -> Product5/1
  Product6/1 -> Fcn1/1
  [u] -> Product2/3
  Signal Specification/1 -> [xe]
  Transpose8/1 -> Product7/1
  Ozone-Gas2/1 -> [W2]
  Transpose10/1 -> Gain3/1
  [xe] -> Product8/2
  Product8/1 -> Fcn4/1
  Product/1 -> Add/1
  Transpose15/1 -> Product12/1
  [xe] -> Product9/2
  Constant8/1 -> Transpose4/1
  [xe] -> Product6/2
  Transpose7/1 -> Product6/1
  [P] -> Product3/2
  Constant9/1 -> Transpose5/1
  Product10/1 -> Fcn5/1
  [xe] -> Product10/2
  [xe] -> Add1/1
  Add/1 -> Ozone-Gas3/1
  [xe] -> Product5/2
  Transpose11/1 -> Gain4/1
  Constant4/1 -> Transpose6/1
  Transpose4/1 -> Product9/1
  Product7/1 -> Fcn2/1
  Product5/1 -> Fcn11/1
  Constant3/1 -> [kw2]
  Constant2/1 -> [kw1]
  Product4/1 -> Ozone-Gas2/1
  Product2/1 -> Add/3
  [Sig] -> Transpose/1
  [A] -> Product/1
  Ozone-Gas1/1 -> [W1]
  Constant/1 -> [A]
  Product1/1 -> Add/2
  [W1] -> Display5/1
  [Delta] -> Transpose16/1
  Transpose16/1 -> Product13/1
  Product13/1 -> Ozone-Gas4/1
  [Delta] -> Product13/2
  Ozone-Gas4/1 -> To File4/1
  [inRev7] -> Vector Concatenate1/1
  [inRev12] -> Vector Concatenate1/4
  Vector Concatenate1/1 -> [inAll]
  [inRev9] -> Vector Concatenate1/2
  [inRev2] -> Vector Concatenate1/3
  [inAll] -> Display6/1
  [Phi] -> Create Diagonal Matrix/1
  Create Diagonal Matrix/1 -> [PhiDiag]
  [Delta] -> Display7/1
  [Delta] -> Create Diagonal Matrix1/1
  Create Diagonal Matrix1/1 -> [DeltaDiag]
  [u] -> Create Diagonal Matrix2/1
  Create Diagonal Matrix2/1 -> [UDiag]
  [UDiag] -> Product4/4
  [PhiDiag] -> Product4/5
  [W2] -> Display8/1
  outAll1/1 -> Mux4/1  "rev7"
  outAll1/4 -> Mux7/1  "rev12"
  Demux2/4 -> Mux7/2
  Demux2/1 -> Mux4/2
  Demux2/2 -> Mux5/2
  outAll1/2 -> Mux5/1  "rev9"
  [xe] -> Demux2/1
  [outAll] -> outAll1/1
  outAll1/3 -> Mux6/1  "rev10"
  Demux2/3 -> Mux6/2
  Log10/1 -> Scope1/1
  Log3/1 -> Scope1/4
  Mux6/1 -> Add Constant2/1
  Log2/1 -> Scope1/3
  Log1/1 -> Scope1/2
  Mux4/1 -> Add Constant/1
  Add Constant/1 -> Log10/1
  Add Constant2/1 -> Log2/1
  Add Constant1/1 -> Log1/1
  Mux5/1 -> Add Constant1/1
  Mux7/1 -> Add Constant3/1
  Add Constant3/1 -> Log3/1
  [outAll] -> Display/1
  Product14/1 -> Fcn8/1
  Transpose1/1 -> Product14/1
  [xe] -> Product14/2
  Constant12/1 -> Transpose1/1
  Product15/1 -> Fcn9/1
  Transpose13/1 -> Product15/1
  [xe] -> Product15/2
  Constant13/1 -> Transpose13/1
  Fcn9/1 -> Vector Concatenate2/6
  Fcn8/1 -> Vector Concatenate2/5
  Constant14/1 -> Transpose17/1
  Product16/1 -> Fcn10/1
  [xe] -> Product16/2
  Transpose17/1 -> Product16/1
  Fcn10/1 -> Vector Concatenate3/5
  Constant15/1 -> Transpose18/1
  Product17/1 -> Fcn12/1
  [xe] -> Product17/2
  Transpose18/1 -> Product17/1
  Fcn12/1 -> Vector Concatenate3/6
  [inRev6] -> Vector Concatenate1/6
  [inRev3] -> Vector Concatenate1/5
  [outRev6] -> Vector Concatenate/6
  [outRev3] -> Vector Concatenate/5
  Constant16/1 -> [Const]
  Matrix Multiply/1 -> [Delta_old]
  Add1/1 -> Matrix Multiply/2
  Constant1/1 -> Matrix Multiply/1
  Demux1/1 -> Mux/2
  " "/2 -> Mux1/1  "rev9"
  " "/1 -> Mux/1  "rev7"
  Demux1/2 -> Mux1/2
  Mux9/1 -> Scope/6
  " "/6 -> Mux9/1  "rev6"
  " "/5 -> Mux8/1  "rev3"
  [outAll] -> " "/1
  Demux1/3 -> Mux2/2
  Mux/1 -> Scope/1
  Mux3/1 -> Scope/4
  Demux1/5 -> Mux8/2
  [xe] -> Demux1/1
  Demux1/4 -> Mux3/2
  Mux8/1 -> Scope/5
  Mux1/1 -> Scope/2
  Demux1/6 -> Mux9/2
  Mux2/1 -> Scope/3
  " "/3 -> Mux2/1  "rev2"
  " "/4 -> Mux3/1  "rev12"
  Clock13/1 -> Fcn25/1
  Fcn25/1 -> [high_b_1]
  Clock14/1 -> Fcn26/1
  Fcn26/1 -> [high_b_2]
  Clock15/1 -> Fcn27/1
  Fcn27/1 -> [high_b_3]
  Clock16/1 -> Fcn28/1
  Clock17/1 -> Fcn29/1
  Clock18/1 -> Fcn30/1
  Fcn30/1 -> [high_b_6]
  Fcn29/1 -> [high_b_5]
  Fcn28/1 -> [high_b_4]
  Clock19/1 -> Fcn31/1
  Fcn31/1 -> [low_b_1]
  Clock20/1 -> Fcn32/1
  Fcn32/1 -> [low_b_2]
  Clock21/1 -> Fcn33/1
  Clock22/1 -> Fcn34/1
  Clock23/1 -> Fcn35/1
  Clock24/1 -> Fcn36/1
  Fcn36/1 -> [low_b_6]
  Fcn35/1 -> [low_b_5]
  Fcn34/1 -> [low_b_4]
  Fcn33/1 -> [low_b_3]
  [high_b_1] -> Mux/3
  [low_b_1] -> Mux/4
  [low_b_2] -> Mux1/4
  [high_b_2] -> Mux1/3
  [low_b_3] -> Mux2/4
  [high_b_3] -> Mux2/3
  [high_b_4] -> Mux3/3
  [low_b_4] -> Mux3/4
  [high_b_5] -> Mux8/3
  [low_b_5] -> Mux8/4
  [high_b_6] -> Mux9/3
  [low_b_6] -> Mux9/4
  [xe] -> Demux3/1
  Constant18/1 -> [eps]
  [Delta_old] -> Demux4/1
  [eps] -> Demux5/1
  projector 1/1(Out1) -> Vector Concatenate4/1
  Demux3/1 -> projector 1/1(In1)
  Demux4/1 -> projector 1/2(In2)
  Demux5/1 -> projector 1/3(In3)
  progector 2/1(Out1) -> Vector Concatenate4/2
  Demux3/2 -> progector 2/1(In1)
  Demux4/2 -> progector 2/2(In2)
  Demux5/2 -> progector 2/3(In3)
  Demux5/6 -> progector 6/3(In3)
  Demux5/5 -> progector 5/3(In3)
  Demux5/4 -> progector 4/3(In3)
  Demux5/3 -> progector 3/3(In3)
  Demux4/6 -> progector 6/2(In2)
  Demux4/5 -> progector 5/2(In2)
  Demux4/4 -> progector 4/2(In2)
  Demux4/3 -> progector 3/2(In2)
  Demux3/3 -> progector 3/1(In1)
  Demux3/4 -> progector 4/1(In1)
  Demux3/5 -> progector 5/1(In1)
  Demux3/6 -> progector 6/1(In1)
  progector 3/1(Out1) -> Vector Concatenate4/3
  progector 4/1(Out1) -> Vector Concatenate4/4
  progector 5/1(Out1) -> Vector Concatenate4/5
  progector 6/1(Out1) -> Vector Concatenate4/6
  [W2] -> Extract Diagonal/1
  Demux6/1 -> Scope14/1
  Demux6/2 -> Scope14/2
  Demux6/3 -> Scope14/3
  Demux6/4 -> Scope14/4
  Demux6/5 -> Scope14/5
  Demux6/6 -> Scope14/6
  Extract Diagonal/1 -> Demux6/1
  Vector Concatenate4/1 -> [Delta]
  connections:
  Transform/LConn1 -- MechanismConfiguration/RConn1 -- Solver Configuration/RConn1 -- World/RConn1
  Revolute/LConn1 -- T501_C_1_RIGID/RConn1
  Revolute4/RConn1 -- T501_C_1_RIGID/LConn1
  Revolute5/LConn1 -- T501_C_6_RIGID/RConn1
  Revolute5/RConn1 -- T501_D_6_RIGID/LConn1
  Revolute6/LConn1 -- T501_D_6_RIGID/RConn1
  Cabina_2_RIGID/LConn1 -- Revolute6/RConn1
  Revolute7/LConn1 -- T403_1_RIGID/RConn1
  Revolute7/RConn1 -- T301_B_1_RIGID/LConn3
  Revolute8/LConn1 -- T301_D_1_RIGID/RConn2
  Revolute8/RConn1 -- T403_1_RIGID/LConn1
  Revolute9/LConn1 -- T301_A_1_RIGID/RConn1
  Revolute/RConn1 -- T501_A_1_RIGID/LConn2
  Revolute9/RConn1 -- T201_A_1_RIGID/LConn2
  Revolute10/LConn1 -- T303_C_1_RIGID/RConn2
  Revolute10/RConn1 -- T301_A_1_RIGID/LConn1
  Revolute11/LConn1 -- T301_E_1_RIGID/RConn1
  Revolute11/RConn1 -- T301_B_1_RIGID/LConn1
  Revolute12/LConn1 -- T303_C_1_RIGID/RConn1
  Revolute12/RConn1 -- T301_B_1_RIGID/LConn2
  Revolute13/LConn1 -- T301_D_1_RIGID/RConn1
  Revolute13/RConn1 -- T303_C_1_RIGID/LConn1
  Revolute14/LConn1 -- T301_F_1_RIGID/RConn1
  Revolute1/LConn1 -- T403_1_RIGID/RConn2
  Revolute14/RConn1 -- T301_E_1_RIGID/LConn1
  T201_A_1_RIGID/LConn1 -- Transform/RConn1
  Revolute1/RConn1 -- T501_A_1_RIGID/LConn1
  Revolute2/LConn1 -- T501_A_6_RIGID/RConn1
  Revolute2/RConn1 -- T501_C_6_RIGID/LConn1
  Revolute3/LConn1 -- T501_D_1_RIGID/RConn2
  Revolute3/RConn1 -- T501_A_6_RIGID/LConn1
  Revolute4/LConn1 -- T501_D_1_RIGID/RConn1
  Subsystem_6/RConn1 -- Revolute6/LConn2
  Revolute6/RConn2 -- Subsystem_6/LConn1
  Subsystem_5/RConn1 -- Revolute5/LConn2
  Revolute5/RConn2 -- Subsystem_5/LConn1
  Subsystem_2/RConn1 -- Revolute2/LConn2
  Subsystem_2/LConn1 -- Revolute2/RConn2
  Subsystem_3/RConn1 -- Revolute3/LConn2
  Subsystem_3/LConn1 -- Revolute3/RConn2
  Subsystem_7/RConn1 -- Revolute7/LConn2
  Subsystem_7/LConn1 -- Revolute7/RConn2
  Subsystem_9/RConn1 -- Revolute9/LConn2
  Subsystem_9/LConn1 -- Revolute9/RConn2
  Subsystem_1/RConn1 -- Revolute1/LConn2
  Subsystem_1/LConn1 -- Revolute1/RConn2
  Subsystem_8/RConn1 -- Revolute8/LConn2
  Subsystem_8/LConn1 -- Revolute8/RConn2
  Subsystem_14/RConn1 -- Revolute14/LConn2
  Subsystem_14/LConn1 -- Revolute14/RConn2
  Subsystem_11/RConn1 -- Revolute11/LConn2
  Subsystem_11/LConn1 -- Revolute11/RConn2
  Subsystem_10/RConn1 -- Revolute10/LConn2
  Subsystem_10/LConn1 -- Revolute10/RConn2
  Subsystem_12/RConn1 -- Revolute12/LConn2
  Subsystem_12/LConn1 -- Revolute12/RConn2
  Subsystem_13/RConn1 -- Revolute13/LConn2
  Subsystem_13/LConn1 -- Revolute13/RConn2
  Subsystem/LConn1 -- Revolute/RConn2
  Subsystem/RConn1 -- Revolute/LConn2
  Subsystem_4/RConn1 -- Revolute4/LConn2
  Subsystem_4/LConn1 -- Revolute4/RConn2

== system DNN_x3D_M_2000iA900L_with_6_rev_21a/Cabina_2_RIGID ==
  ReferenceFrame : sm_lib/Frames and Transforms/Reference Frame
  Solid : sm_lib/Body Elements/File Solid  ExtGeomFileName=Cabina_Predeterminado_sldprt.STEP  UnitType=FromFile  ExtGeomFileUnits=m  StepReaderType=HEX  ExportConvexHullGeometry=off  InertiaType=Custom  Mass=smiData.Solid(2).mass  MassUnits=kg  CenterOfMass=smiData.Solid(2).CoM  CenterOfMassUnits=cm  MomentsOfInertia=smiData.Solid(2).MoI  MomentsOfInertiaUnits=kg*cm^2  ProductsOfInertia=smiData.Solid(2).PoI  ProductsOfInertiaUnits=kg*cm^2  BasedOnType=DensityFromFile  Density=1000  DensityUnits=kg/m^3  DoExposeReferenceFrame=on  SerializedFrames=<Frames/>  GraphicType=FromGeometry  MarkerShape=Sphere  MarkerSize=10  GraphicVisPropType=SimpleVisualProperties  GraphicDiffuseColor=smiData.Solid(2).color  GraphicSpecularColor=[0.5 0.5 0.5 1.0]  GraphicAmbientColor=[0.15 0.15 0.15 1.0]  GraphicEmissiveColor=[0.0 0.0 0.0 1.0]  GraphicShininess=75  GraphicOpacity=smiData.Solid(2).opacity
  Transform : sm_lib/Frames and Transforms/Rigid Transform  TranslationMethod=Cartesian  TranslationStandardOffset=0  TranslationLengthUnit=mm  TranslationStandardAxis=+Z  TranslationCartesianOffset=smiData.RigidTransform(14).translation  TranslationROffset=0  TranslationROffsetUnits=m  TranslationZOffset=0  TranslationZOffsetUnits=m  TranslationThetaOffset=0  TranslationThetaOffsetUnits=deg  RotationMethod=ArbitraryAxis  RotationAngleUnits=rad  RotationStandardAxis=+Z  RotationAngle=smiData.RigidTransform(14).angle  RotationArbitraryAxis=smiData.RigidTransform(14).axis  FollAlignAxisA=+X  BaseAlignAxisA=+Y  FollAlignAxisB=+Y  BaseAlignAxisB=+Z  RotationSequenceAxes=FollowerAxes  RotationSequence=XYX  RotationSequenceAngles=[0 0 0]  RotationSequenceAnglesUnits=deg  RotationMatrix=[1 0 0; 0 1 0; 0 0 1]
  F : PMIOPort  Side=Left
  connections:
  Solid/RConn1 -- ReferenceFrame/RConn1 -- Transform/LConn1
  Transform/RConn1 -- F/RConn1

== system DNN_x3D_M_2000iA900L_with_6_rev_21a/Subsystem ==
  Add5 : Sum  Inputs=-+
  Constant6 : Constant  Value=0
  PID Controller5 : pid_lib/PID Controller  Controller=PID  Form=Parallel  TimeDomain=Continuous-time  UseExternalTs=off  SampleTime=-1  IntegratorMethod=Forward Euler  FilterMethod=Forward Euler  ControllerParametersSource=internal  P=450  I=150  D=1400  N=100  UseFilter=on  TunerSelectOption=Transfer Function Based (PID Tuner App)  InitialConditionSource=internal  InitialConditionForIntegrator=0  InitialConditionForFilter=0  DifferentiatorICPrevScaledInput=0  ExternalReset=none  TrackingMode=off  Kt=1  LimitOutput=off  SatLimitsSource=internal  UpperSaturationLimit=inf  LowerSaturationLimit=-inf  LinearizeAsGain=on  AntiWindupMode=none  Kb=1  POutMin=[]  POutMax=[]  IOutMin=[]  IOutMax=[]  DOutMin=[]  DOutMax=[]  NOutMin=[]  NOutMax=[]  SumOutMin=[]  SumOutMax=[]  SaturationOutMin=[]  SaturationOutMax=[]  PParamMin=[]  PParamMax=[]  IParamMin=[]  IParamMax=[]  DParamMin=[]  DParamMax=[]  NParamMin=[]  NParamMax=[]  KbParamMin=[]  KbParamMax=[]  KtParamMin=[]  KtParamMax=[]  KbOutMin=[]  KbOutMax=[]  KtOutMin=[]  KtOutMax=[]  IntegratorOutMin=[]  IntegratorOutMax=[]  FilterOutMin=[]  FilterOutMax=[]  SumI1OutMin=[]  SumI1OutMax=[]  SumI2OutMin=[]  SumI2OutMax=[]  SumI3OutMin=[]  SumI3OutMax=[]  SumI4OutMin=[]  SumI4OutMax=[]  SumDOutMin=[]  SumDOutMax=[]  DifferentiatorOutMin=[]  DifferentiatorOutMax=[]  FilterDiffOutCoefMin=[]  FilterDiffOutCoefMax=[]  ReciprocalOutMin=[]  ReciprocalOutMax=[]  SumDenOutMin=[]  SumDenOutMax=[]  SumNumOutMin=[]  SumNumOutMax=[]  DivideOutMin=[]  DivideOutMax=[]  UdiffTsProdOutMin=[]  UdiffTsProdOutMax=[]  NTsProdOutMin=[]  NTsProdOutMax=[]  UintegralTsProdOutMin=[]  UintegralTsProdOutMax=[]  UngainTsProdOutMin=[]  UngainTsProdOutMax=[]  IntegratorContinuousStateAttributes=''  IntegratorStateMustResolveToSignalObject=off  IntegratorRTWStateStorageClass=Auto  FilterContinuousStateAttributes=''  FilterStateMustResolveToSignalObject=off  FilterRTWStateStorageClass=Auto  ParallelPVariant=InternalParameters  IdealPVariant=Disabled  IVariant=InternalParameters  DVariant=InternalParameters  IntegratorVariant=Continuous  SatVariant=Disabled  AWVariant=Passthrough  PCopyVariant=Disabled  TRVariant=Disabled  FdbkBlocksVariant=Forward  IdealPFdbkVariant=Disabled  SatFdbkVariant=Disabled  DerivativeFilterVariant=ContFilter  NVariant=InternalParameters  NCopyVariant=Disabled  FilterICVariant=InternalICsFilter  IntegratorICVariant=InternalICs  ExternalResetVariant=Disabled  TRSumVariant=Passthrough  SumFdbkVariant=Disabled  SumVariant=Sum_PID  TsampFilterVariant=InternalTs  TsampNgainVariant=Passthrough  TsampIntegralVariant=Passthrough  ExternalSaturationOutDataTypeStr=Inherit: Same as second input
  PS-Simulink Converter5 : nesl_utility/PS-Simulink Converter  PhysicalDomain=network_engine_domain  SubClassName=ps_output  LeftPortType=input  RightPortType=output  PseudoPeriodic=off  Frequencies=[]  VectorFormat=1-D array  Unit=inherit  AffineConversion=off
      settings: SourceProductBaseCode=SS,PW,VE
  Scope5 : Scope  NumInputPorts=2
  Simulink-PS Converter5 : nesl_utility/Simulink-PS Converter  PhysicalDomain=network_engine_domain  SubClassName=ps_input  LeftPortType=input  RightPortType=output  PseudoPeriodic=off  Frequencies=[]  NoiseDistribution=none  NoiseParameters=[]  Unit=1  AffineConversion=off  FilteringAndDerivatives=provide  SimscapeFilterOrder=1  InputFilterTimeConstant=0.001  UdotUserProvided=0
      settings: SourceProductBaseCode=SS,PW,VE
  output : PMIOPort  Side=Right
  input : PMIOPort  Port=2  Side=Left
  wires:
  PID Controller5/1 -> Simulink-PS Converter5/1
  Add5/1 -> PID Controller5/1
  Constant6/1 -> Scope5/1, Add5/2
  PS-Simulink Converter5/1 -> Add5/1, Scope5/2
  connections:
  Simulink-PS Converter5/RConn1 -- output/RConn1
  PS-Simulink Converter5/LConn1 -- input/RConn1
